simulink model "lander_sim_complex"  (R2023a)
settings: Solver=VariableStepAuto  StartTime=0.0  StopTime=10.0  RelTol=1e-3
libraries: simulink x1
settings Model: Creator=User  LastModifiedBy=User

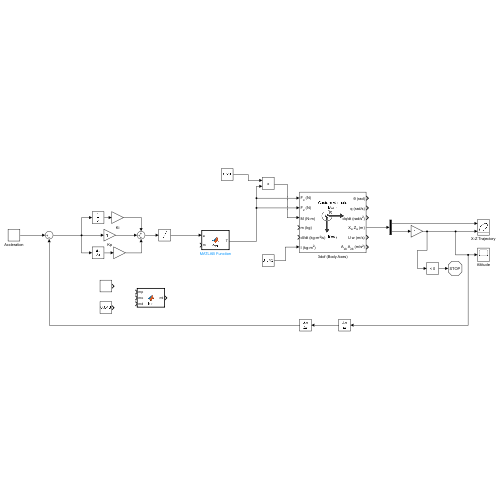
[thumbnail: Simulink's stored preview of the top-level diagram]
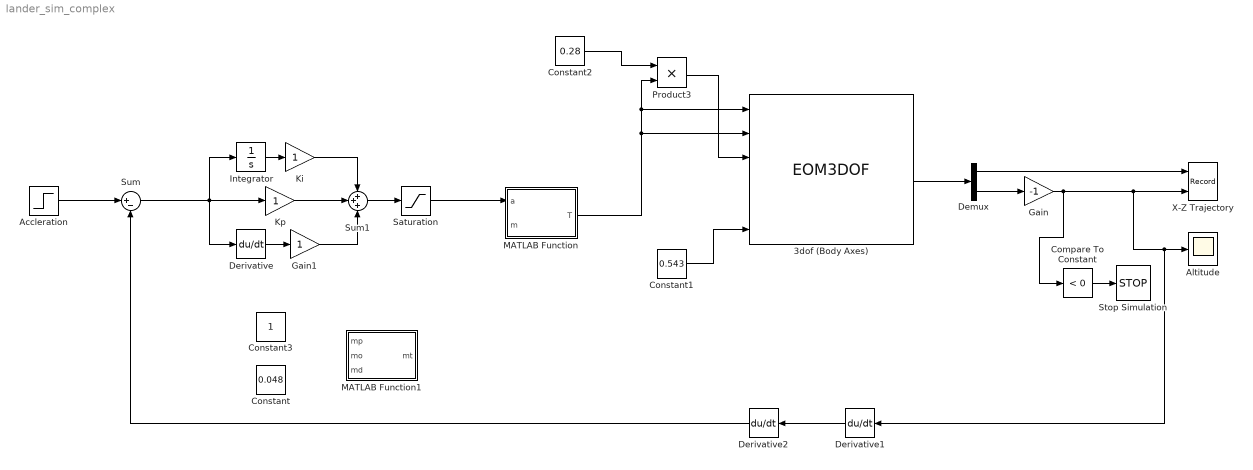
== system lander_sim_complex ==
  3dof (Body Axes) : EOM3DOF  mtype=Custom Variable  v_ini=0  mass=0.543  Iyy=0.048
  Accleration : Step  Time=2  Before=-312.5  After=0  SampleTime=0
  Altitude : Scope
  Compare To Constant : simulink/Logic and Bit Operations/Compare To Constant  relop=<  const=0  OutDataTypeStr=boolean
  Constant : Constant  Value=0.048
  Constant1 : Constant  Value=0.543
  Constant2 : Constant  Value=0.28
  Constant3 : Constant
  Demux : Demux  Outputs=2
  Derivative : Derivative
  Derivative1 : Derivative
  Derivative2 : Derivative
  Gain : Gain  Gain=-1
  Gain1 : Gain
  Integrator : Integrator
  Ki : Gain
  Kp : Gain
  MATLAB Function : MATLAB Function  TreatAsAtomicUnit=on
  MATLAB Function1 : MATLAB Function  TreatAsAtomicUnit=on
  Product3 : Product
  Saturation : Saturate  UpperLimit=7  LowerLimit=-7
  Stop Simulation : Stop
  Sum : Sum  Inputs=|+-
  Sum1 : Sum  Inputs=+++
  X-Z Trajectory : Record  FileSettingsInternal="{\"entries\":[{\"content\":{\"excelSettings\":{\"content\":{},\"type\":\"Streamout.ExcelSettings\"}},\"type\":\"Streamout.FileSettingStorage\",\"uuid\":\"a9713351-d3f8-4cdd-bdcf-73c13cfacd61\"}],\"packageUris\":[\"http://schema.mathworks.com/mf0/streamout_blocks/R2020a\"],\"version\":\"1.0\"}"  Layout=[1 1]  SignalsInternal="{\"entries\":[{\"content\":{\"signals\":[{\"content\":{\"blockPath\":[\"lander_sim_complex/X-Z Trajectory\"],\"dimensions\":[1],\"domain\":\"lander_sim_complex/X-Z Trajectory\",\"lineColor\":\"#a2142f\",\"plots\":[1],\"port\":1,\"signalID\":8,\"signalName\":\"Demux:1\"},\"type\":\"RecordBlkView.Signal\",\"uuid\":\"e5ab0f89-3053-4d97-82af-9ae4bf729244\"},{\"content\":{\"blockPath\":[\"lander_sim_complex/X-Z Trajectory\"],\"dimensions\":[1],\"domain\":\"lander_sim_complex/X-Z Trajectory\",\"lineColor\":\"#139fff\",\"plots\":[1],\"port\":2,\"signalID\":11,\"signalName\":\"Gain\"},\"type\":\"RecordBlkView.Signal\",\"uuid\":\"b5c8c16e-af58-4736-a330-edf39468cc9e\"}]},\"type\":\"RecordBlkView.InputSignals\",\"uuid\":\"6ffeb9bb-22ac-469e-bb5a-19220f649136\"}],\"packageUris\":[\"http://schema.mathworks.com/mf0/streamout_blocks/R2020a\"],\"version\":\"1.0\"}"  VisualizationBindings="{\"xyplotplugin\":{\"info\":[{\"series\":[{\"bindingParametersList\":[{\"parameter\":\"X-Axis\",\"signalID\":8,\"signalName\":\"Demux:1\"},{\"parameter\":\"Y-Axis\",\"signalID\":11,\"signalName\":\"Gain\"}],\"seriesID\":24736}],\"subplotID\":1}]}}"  CompatibilityTag=XY  st=-1
  wires:
  Compare To Constant/1 -> Stop Simulation/1
  Demux/2 -> Gain/1
  Gain/1 -> Compare To Constant/1, Derivative1/1, Altitude/1, X-Z Trajectory/2
  3dof (Body Axes)/4 -> Demux/1
  Demux/1 -> X-Z Trajectory/1
  Sum/1 -> Derivative/1, Integrator/1, Kp/1
  Integrator/1 -> Ki/1
  Ki/1 -> Sum1/1
  Kp/1 -> Sum1/2
  Derivative/1 -> Gain1/1
  Gain1/1 -> Sum1/3
  Accleration/1 -> Sum/1
  Sum1/1 -> Saturation/1
  Derivative2/1 -> Sum/2
  MATLAB Function/1(T) -> 3dof (Body Axes)/1, Product3/2, 3dof (Body Axes)/2
  Saturation/1 -> MATLAB Function/1(a)
  Constant1/1 -> 3dof (Body Axes)/6
  Constant2/1 -> Product3/1
  Product3/1 -> 3dof (Body Axes)/3
  Derivative1/1 -> Derivative2/1

== matlab function lander_sim_complex/MATLAB Function ==
  data: a input; T output; m input
function T = fcn(a, m)

T = m*a;

== matlab function lander_sim_complex/MATLAB Function1 ==
  data: mp input; mt output; mo input; md input
function mt = fcn(mp, mo, md)

mt = mp+mo+md;
